simulink library "lib_Convection_FCHorizRectCavity"  (R2015a)
settings: Solver=ode45  StartTime=0.0  StopTime=10.0  RelTol=1e-3
libraries: simulink x2
settings Model: Creator=jlkratz  LastModifiedBy=jlkratz

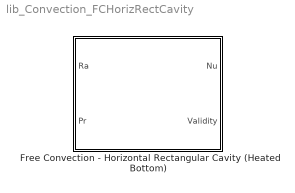
== system lib_Convection_FCHorizRectCavity ==
  Free Convection - Horizontal Rectangular Cavity (Heated Bottom) : Subsystem  mask(TSAT: Horizontal Rectangular Cavity (Heated Bottom)){}
      mask help:
      | This block gives first approximation of the average Nusselt number of free convection within a horizontal cavity with the bottom side heated. Note that all fluid properrties should be evaluated at average of the hot and cold surface. Also note that the charateristic length used to calculate the Rayleigh number should be the distance between the hot and cold surfaces (L). The correlation employed was recommended by Globe and Dropkin and applies for values of L/H that are sufficiently small such that the effects of the side walls are negligible. The variable H refers to the wdith of the horizontal cavity. The correlation is valide for the following conditions:
      |
      | 300000 <= Ra <= 7*10^9
      |
      | Note that for the case when the heated surface is on top, the heat transfer from the top to the bottom surface is exclusively by conduction (Nu = 1), in the absence of radiation. This result is irrespective of the value of the Rayliegh number. See the block help menu for more information.
      mask Help: web(which('Convection_TSAT_FCHorizRectCavity.html'),'-helpbrowser')

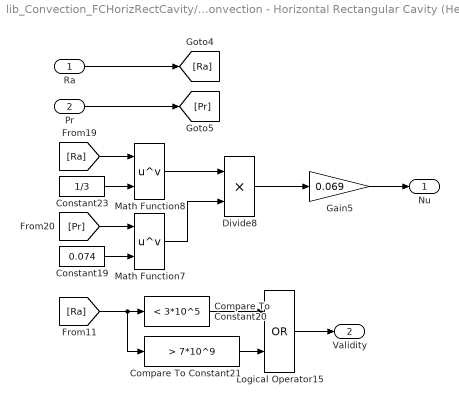
== system lib_Convection_FCHorizRectCavity/Free Convection - Horizontal Rectangular Cavity (Heated Bottom) ==
  Ra : Inport
  Pr : Inport  Port=2
  Compare To Constant20 : simulink/Logic and Bit Operations/Compare To Constant  relop=<  const=3*10^5  OutDataTypeStr=boolean
  Compare To Constant21 : simulink/Logic and Bit Operations/Compare To Constant  relop=>  const=7*10^9  OutDataTypeStr=boolean
  Constant19 : Constant  Value=0.074
  Constant23 : Constant  Value=1/3
  Divide8 : Product  Inputs=**
  Gain5 : Gain  Gain=0.069
  Logical Operator15 : Logic  Operator=OR  AllPortsSameDT=off  OutDataTypeStr=boolean
  Math Function7 : Math  Operator=pow  SaturateOnIntegerOverflow=on
  Math Function8 : Math  Operator=pow  SaturateOnIntegerOverflow=on
  Nu : Outport
  Validity : Outport  Port=2
  wires:
  Logical Operator15/1 -> Validity/1
  Gain5/1 -> Nu/1
  Divide8/1 -> Gain5/1
  Math Function7/1 -> Divide8/2
  Math Function8/1 -> Divide8/1
  Constant23/1 -> Math Function8/2
  [Ra] -> Math Function8/1
  Constant19/1 -> Math Function7/2
  [Pr] -> Math Function7/1
  Compare To Constant21/1 -> Logical Operator15/2
  Compare To Constant20/1 -> Logical Operator15/1
  [Ra] -> Compare To Constant21/1, Compare To Constant20/1
  Pr/1 -> [Pr]
  Ra/1 -> [Ra]
